simulink model "direct_event1_eg_4"  (R2018a)
settings: Solver=VariableStepAuto  StartTime=0.0  StopTime=10.0  RelTol=1e-3
settings Model: Creator=86188  LastModifiedBy=86188

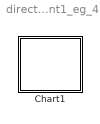
== system direct_event1_eg_4 ==
  Chart1 : Stateflow chart  TreatAsAtomicUnit=on

== stateflow chart direct_event1_eg_4/Chart1 ==
  settings: executeAtInitialization=1
  state A
  state B
  state C
    state C1
    state C2
    (default) -> C1
    C1 -> C2 : F
  (default) -> A
  A -> B [order 1] : [data==1]{data=2;send(F,A);}
  A -> C [order 2] : F
  data: M local; data local =1
  events: F local FUNCTION_CALL_EVENT
